simulink model "Cruise_Model_V16"  (R2024a)
settings: Solver=ode23t  StartTime=0.0  StopTime=t5(end)  RelTol=1e-3
values from neighbouring files (symbols this model uses):
  coefficients =     [UAM2.mat]    (also in VX4_cur.mat; VX4data.mat; alexisignoringme11UAM2.mat; alexisignoringme12.mat)
  idxf = [1 78 155 231 308 385 462 538 615 692 769 845 ... (70 elements, 1x70)]    [alexisignoringme.mat]    (also in alexisignoringme11UAM2.mat = [1 112 223 334 445 555 666 777 888 999 1001 1112 ... (50 ele; alexisignoringme12.mat = [1 54 106 159 211 264 316 369 421 474 526 579 ... (100 eleme; alexisignoringme13.mat = [1 54 106 159 211 264 316 369 421 474 526 579 ... (100 eleme; alexisignoringme14.mat = [1 500 999 1001 1500 1999 2001 2500 2999 3001 3500 3999 ... )
  Kpi = lqr(sys, Q, R)    [QRerr_LQI.m]    (also in alexisignoringme8.mat = [9.62344892608e-17 -1.21933000029e-16 1.4312558077e-15 29.45)
  missionruntime =     [alexisignoringme4.mat]    (also in alexisignoringme5.mat; alexisignoringme6.mat; alexisignoringme7.mat; alexisignoringme8.mat)
  q = 0.5*1.225*airflow.U^2    [VLMV3.m]    (also in VLMV3_modified.m = 0.5*1.225*airflow.U^2*Sref)
  Ut = [0 0 -4.89661324026e-08 0 0 -1504.57476188 -0.000428335964898 -1.57410795509e-09 3.42121377805e-06 0 0 0 ... (450 elements, 9x50)]    [alexisignoringme5.mat]    (also in alexisignoringme6.mat; alexisignoringme7.mat; alexisignoringme8.mat = [0 0 0 0 0 -1498.96331992 -4.41873387445e-05 -1.31180695462e)
  uvec = [0.1 3.42222222222 6.74444444444 10.0666666667 13.3888888889 16.7111111111 20.0333333333 23.3555555556 26.6777777778 30]    [alexisignoringme.mat]    (also in alexisignoringme4.mat; alexisignoringme5.mat; alexisignoringme6.mat; alexisignoringme7.mat)
  X = [0.00351660116596 0 -9.99999602467 0 0 0 2.75026701025e-08 -4.1982332666e-06 -1.5333765693e-08 0.000503097278932 0 -6.54626389426e-11 ... (630 elements, 9x5x14)]    [alexisignoringme.mat]    (also in alexisignoringme12.mat = [0.000256495736971 0 -9.99999647184 0 0 0 0 -3.73764411116e-; alexisignoringme13.mat = [0.00833666803911 0 -10.0000021435 0 0 0 0 7.14203458163e-06; alexisignoringme14.mat = [0.00833666803911 0 -10.0000021435 0 0 0 0 7.14203458163e-06; alexisignoringme4.mat = [0.00351658839646 0 -9.99999599468 0 0 0 2.7327442949e-09 -4)
  Xes = X(:,idx(4))    [QRerr_LQI.m]    (also in QRerr_p.m = X(:,idx(2)); alexisignoringme4.mat = [0.00351658839646 0 -9.99999599468 0 0 0 2.7327442949e-09 -4; alexisignoringme5.mat = [0 0 -1.11199998303 0 0 0 -1.38069247376e-09 1.48137256273e-; alexisignoringme6.mat = [0 0 -1.11199998303 0 0 0 -1.38069247376e-09 1.48137256273e-)
undefined symbols (not defined in the file or in its folder): F, Light, MIL, tl, VX4, xvec
libraries: slpidlib x14, aerolibwind2 x8, aerolibatmos2 x4, shared6dof x1
(part 3 of 3)

== system Cruise_Model_V16/Trim Solver and Actuation/Controller/Trim Solver/Back-calculation ==
  et : Inport
  Gain : Gain  Gain=2
  Transpose : Math  Operator=transpose
  Out1 : Outport
  wires:
  Gain/1 -> Transpose/1
  et/1 -> Gain/1
  Transpose/1 -> Out1/1

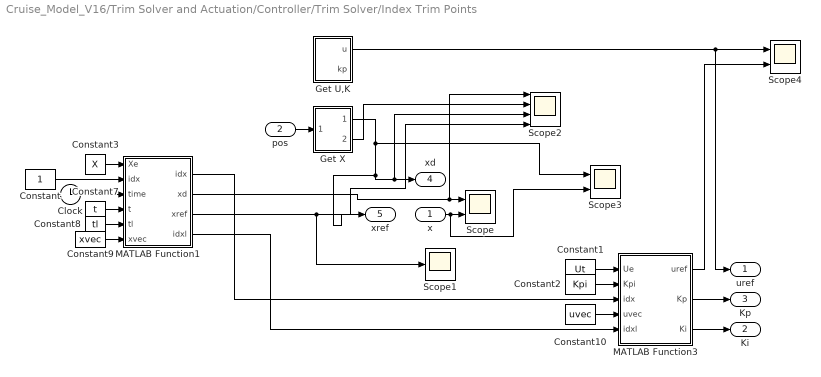
== system Cruise_Model_V16/Trim Solver and Actuation/Controller/Trim Solver/Index Trim Points ==
  x : Inport
  pos : Inport  Port=2
  Clock : Clock
  Constant : Constant
  Constant1 : Constant  Value=Ut
  Constant10 : Constant  Value=uvec
  Constant2 : Constant  Value=Kpi
  Constant3 : Constant  Value=X
  Constant7 : Constant  Value=t
  Constant8 : Constant  Value=tl
  Constant9 : Constant  Value=xvec
  Get U,K : Subsystem
  Get X : Subsystem
  MATLAB Function1 : MATLAB Function  InitFcn=load buses.mat  StartFcn=load buses.mat  TreatAsAtomicUnit=on  VariantControl=Choice
      settings: OpenFcn=load buses.mat
  MATLAB Function3 : MATLAB Function  InitFcn=load buses.mat  StartFcn=load buses.mat  TreatAsAtomicUnit=on  VariantControl=Choice
      settings: OpenFcn=load buses.mat
  Scope : Scope  NumInputPorts=2
  Scope1 : Scope
  Scope2 : Scope  NumInputPorts=4
  Scope3 : Scope  NumInputPorts=2
  Scope4 : Scope  NumInputPorts=2
  uref : Outport
  Ki : Outport  Port=2
  Kp : Outport  Port=3
  xd : Outport  Port=4
  xref : Outport  Port=5
  wires:
  Constant2/1 -> MATLAB Function3/2(Kpi)
  Constant1/1 -> MATLAB Function3/1(Ue)
  Constant3/1 -> MATLAB Function1/1(Xe)
  MATLAB Function3/1(uref) -> Scope4/2
  Constant8/1 -> MATLAB Function1/5(tl)
  Constant10/1 -> MATLAB Function3/4(uvec)
  MATLAB Function1/4(idxl) -> MATLAB Function3/5(idxl)
  MATLAB Function3/2(Kp) -> Kp/1
  Constant9/1 -> MATLAB Function1/6(xvec)
  Clock/1 -> MATLAB Function1/3(time)
  Constant7/1 -> MATLAB Function1/4(t)
  x/1 -> Scope3/2, Scope/2
  MATLAB Function3/3(Ki) -> Ki/1
  Constant/1 -> MATLAB Function1/2("idx ")
  MATLAB Function1/1(idx) -> MATLAB Function3/3(idx)
  MATLAB Function1/3(xref) -> Scope2/4, Scope1/1
  MATLAB Function1/2(xd) -> Scope2/1, Scope/1
  Get X/1(xref) -> xref/1, Scope2/3, xd/1, Scope3/1
  Get X/2(xd) -> Scope2/2
  Get U,K/1(u) -> uref/1, Scope4/1
  pos/1 -> Get X/1(pos)

== system Cruise_Model_V16/Trim Solver and Actuation/Controller/Trim Solver/Saturation1 ==
  In1 : Inport
  Constant : Constant  Value=0
  Demux3 : Demux  Outputs=9
  Mux : Mux  Inputs=9
  Saturation : Saturate  UpperLimit=0.55  LowerLimit=-0.55
  Saturation1 : Saturate  UpperLimit=0.55  LowerLimit=-0.55
  Saturation2 : Saturate  UpperLimit=0.55  LowerLimit=-0.55
  Saturation3 : Saturate  UpperLimit=1.6*max(abs(Ut(4,:)))  LowerLimit=0
  Saturation4 : Saturate  UpperLimit=0  LowerLimit=-1.6*max(abs(Ut(6,:)))
  Saturation5 : Saturate  UpperLimit=1.6*max(abs(Ut(6,:)))  LowerLimit=-1.6*max(abs(Ut(6,:)))
  Saturation6 : Saturate  UpperLimit=1.6*max(abs(Ut(6,:)))  LowerLimit=-1.6*max(abs(Ut(6,:)))
  Saturation7 : Saturate  UpperLimit=1.6*max(abs(Ut(6,:)))  LowerLimit=-1.6*max(abs(Ut(6,:)))
  Scope : Scope  NumInputPorts=2
  Out1 : Outport
  wires:
  Saturation7/1 -> Mux/9
  Saturation6/1 -> Mux/8
  Saturation5/1 -> Mux/7
  Saturation4/1 -> Mux/6
  Saturation3/1 -> Mux/4
  Saturation2/1 -> Mux/3
  Saturation1/1 -> Mux/2
  Saturation/1 -> Mux/1
  Demux3/9 -> Saturation7/1
  Constant/1 -> Mux/5
  Demux3/8 -> Saturation6/1
  Demux3/7 -> Saturation5/1
  Demux3/6 -> Saturation4/1
  Demux3/4 -> Saturation3/1
  In1/1 -> Demux3/1
  Mux/1 -> Out1/1
  Demux3/1 -> Saturation/1
  Demux3/2 -> Saturation1/1
  Demux3/3 -> Saturation2/1

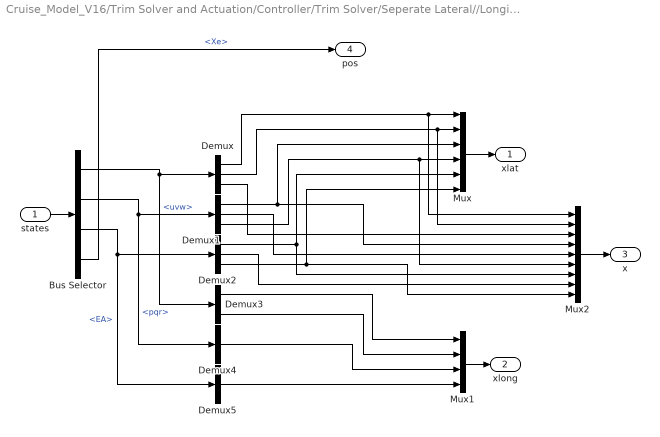
== system Cruise_Model_V16/Trim Solver and Actuation/Controller/Trim Solver/Seperate Lateral//Longitudinal ==
  states : Inport
  Bus Selector : BusSelector  OutputSignals=uvw,pqr,EA,Xe
  Demux{,1..5} (6 alike) : Demux  Outputs=3
  Mux : Mux  Inputs=6
  Mux1 : Mux
  Mux2 : Mux  Inputs=9
  xlat : Outport
  xlong : Outport  Port=2
  x : Outport  Port=3
  pos : Outport  Port=4
  wires:
  states/1 -> Bus Selector/1
  Mux/1 -> xlat/1
  Mux1/1 -> xlong/1
  Bus Selector/1 -> Demux/1, Demux3/1  "<uvw>"
  Bus Selector/2 -> Demux1/1, Demux4/1  "<pqr>"
  Bus Selector/3 -> Demux5/1, Demux2/1  "<EA>"
  Demux/1 -> Mux2/1, Mux/1
  Demux/2 -> Mux2/2, Mux/2
  Demux1/1 -> Mux2/4, Mux/3
  Demux1/3 -> Mux2/6, Mux/4
  Demux2/1 -> Mux2/7, Mux/5
  Demux2/3 -> Mux2/9, Mux/6
  Demux3/1 -> Mux1/1
  Demux3/3 -> Mux1/2
  Demux4/2 -> Mux1/3
  Demux5/2 -> Mux1/4
  Mux2/1 -> x/1
  Demux/3 -> Mux2/3
  Demux1/2 -> Mux2/5
  Demux2/2 -> Mux2/8
  Bus Selector/4 -> pos/1  "<Xe>"

== system Cruise_Model_V16/Trim Solver and Actuation/Controller/Trim Solver/State Passthr. ==
  In2 : Inport
  Demux3 : Demux  Outputs=9
  Mux3 : Mux  Inputs=6
  Terminator : Terminator
  Terminator1 : Terminator
  Terminator2 : Terminator
  Out4 : Outport
  wires:
  Demux3/1 -> Mux3/1
  Demux3/8 -> Mux3/5
  Demux3/7 -> Mux3/4
  Demux3/9 -> Mux3/6
  Demux3/3 -> Mux3/3
  Demux3/2 -> Mux3/2
  Mux3/1 -> Out4/1
  In2/1 -> Demux3/1
  Demux3/4 -> Terminator/1
  Demux3/5 -> Terminator1/1
  Demux3/6 -> Terminator2/1

== system Cruise_Model_V16/Trim Solver and Actuation/Controller/PID_GBDP_withThrust/Altitude Control Path/Step demand for testing ==
  In1 : Inport
  Mux1 : Mux  Inputs=2
  Scope2 : Scope
  Scope4 : Scope
  Step1 : Step  Time=60  Before=-500  After=-490  SampleTime=0
  Step2 : Step  Time=80  After=-10  SampleTime=0
  Step3 : Step  Time=120  After=20  SampleTime=0
  Step4 : Step  Time=120  After=20  SampleTime=0
  Sum : Sum  Inputs=++++
  To Workspace : ToWorkspace  VariableName=altitudeResponse  SaveFormat=Timeseries  SampleTime=-1
  Out1 : Outport
  wires:
  Step3/1 -> Sum/3
  Mux1/1 -> To Workspace/1, Scope4/1
  Sum/1 -> Out1/1, Mux1/1
  Step4/1 -> Sum/4
  Step1/1 -> Sum/1
  In1/1 -> Mux1/2, Scope2/1
  Step2/1 -> Sum/2

== system Cruise_Model_V16/Trim Solver and Actuation/Controller/PID_GBDP_withThrust/Course Angle Control Path/Step demand for testing2 ==
  Va : Inport
  Mux1 : Mux  Inputs=2
  Scope2 : Scope
  Scope4 : Scope
  Step1 : Step  Time=60  Before=0.1  After=0.2  SampleTime=0
  Step2 : Step  Time=80  After=-0.4  SampleTime=0
  Step3 : Step  Time=120  After=-0.2  SampleTime=0
  Step4 : Step  Time=100  After=0.6  SampleTime=0
  Step5 : Step  Time=140  After=-0.4  SampleTime=0
  Sum : Sum  Inputs=+++++
  To Workspace : ToWorkspace  VariableName=headingAngleResponse  SaveFormat=Timeseries  SampleTime=-1
  Out1 : Outport
  wires:
  Step5/1 -> Sum/5
  Step3/1 -> Sum/3
  Mux1/1 -> To Workspace/1, Scope4/1
  Sum/1 -> Out1/1, Mux1/1
  Step4/1 -> Sum/4
  Step1/1 -> Sum/1
  Va/1 -> Mux1/2, Scope2/1
  Step2/1 -> Sum/2

== system Cruise_Model_V16/Trim Solver and Actuation/Controller/PID_GBDP_withThrust/Subsystem/Step demand for testing1 ==
  Va : Inport
  Mux1 : Mux  Inputs=2
  Scope2 : Scope
  Scope4 : Scope
  Step1 : Step  Time=60  Before=25  After=31  SampleTime=0
  Step2 : Step  Time=80  After=-3  SampleTime=0
  Step3 : Step  Time=120  After=-5  SampleTime=0
  Step4 : Step  Time=100  After=8  SampleTime=0
  Step5 : Step  Time=140  After=-2  SampleTime=0
  Sum : Sum  Inputs=+++++
  To Workspace : ToWorkspace  VariableName=airspeedResponse  SaveFormat=Timeseries  SampleTime=-1
  Out1 : Outport
  wires:
  Step2/1 -> Sum/2
  Va/1 -> Scope2/1, Mux1/2
  Step1/1 -> Sum/1
  Step4/1 -> Sum/4
  Sum/1 -> Mux1/1, Out1/1
  Mux1/1 -> Scope4/1, To Workspace/1
  Step3/1 -> Sum/3
  Step5/1 -> Sum/5

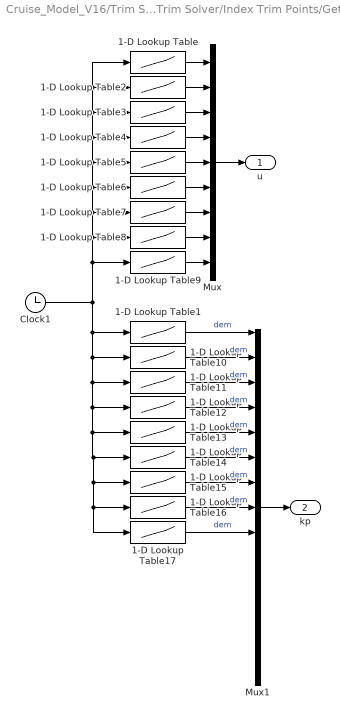
== system Cruise_Model_V16/Trim Solver and Actuation/Controller/Trim Solver/Index Trim Points/Get U,K ==
  1-D Lookup Table : Lookup_n-D  NumberOfTableDimensions=1  BreakpointsForDimension1=t  Table=Ut(1,:)  InternalRulePriority=Speed  RndMeth=Simplest
  1-D Lookup Table1 : Lookup_n-D  NumberOfTableDimensions=1  BreakpointsForDimension1=t(1:end-1)  Table=X(1,2:end)  InternalRulePriority=Speed  RndMeth=Simplest
  1-D Lookup Table10 : Lookup_n-D  NumberOfTableDimensions=1  BreakpointsForDimension1=t(1:end-1)  Table=X(2,2:end)  InternalRulePriority=Speed  RndMeth=Simplest
  1-D Lookup Table11 : Lookup_n-D  NumberOfTableDimensions=1  BreakpointsForDimension1=t(1:end-1)  Table=X(3,2:end)  InternalRulePriority=Speed  RndMeth=Simplest
  1-D Lookup Table12 : Lookup_n-D  NumberOfTableDimensions=1  BreakpointsForDimension1=t(1:end-1)  Table=X(4,2:end)  InternalRulePriority=Speed  RndMeth=Simplest
  1-D Lookup Table13 : Lookup_n-D  NumberOfTableDimensions=1  BreakpointsForDimension1=t(1:end-1)  Table=X(5,2:end)  InternalRulePriority=Speed  RndMeth=Simplest
  1-D Lookup Table14 : Lookup_n-D  NumberOfTableDimensions=1  BreakpointsForDimension1=t(1:end-1)  Table=X(6,2:end)  InternalRulePriority=Speed  RndMeth=Simplest
  1-D Lookup Table15 : Lookup_n-D  NumberOfTableDimensions=1  BreakpointsForDimension1=t(1:end-1)  Table=X(7,2:end)  InternalRulePriority=Speed  RndMeth=Simplest
  1-D Lookup Table16 : Lookup_n-D  NumberOfTableDimensions=1  BreakpointsForDimension1=t(1:end-1)  Table=X(8,2:end)  InternalRulePriority=Speed  RndMeth=Simplest
  1-D Lookup Table17 : Lookup_n-D  NumberOfTableDimensions=1  BreakpointsForDimension1=t(1:end-1)  Table=X(9,2:end)  InternalRulePriority=Speed  RndMeth=Simplest
  1-D Lookup Table2 : Lookup_n-D  NumberOfTableDimensions=1  BreakpointsForDimension1=t  Table=Ut(2,:)  InternalRulePriority=Speed  RndMeth=Simplest
  1-D Lookup Table3 : Lookup_n-D  NumberOfTableDimensions=1  BreakpointsForDimension1=t  Table=Ut(3,:)  InternalRulePriority=Speed  RndMeth=Simplest
  1-D Lookup Table4 : Lookup_n-D  NumberOfTableDimensions=1  BreakpointsForDimension1=t  Table=Ut(4,:)  InternalRulePriority=Speed  RndMeth=Simplest
  1-D Lookup Table5 : Lookup_n-D  NumberOfTableDimensions=1  BreakpointsForDimension1=t  Table=Ut(5,:)  InternalRulePriority=Speed  RndMeth=Simplest
  1-D Lookup Table6 : Lookup_n-D  NumberOfTableDimensions=1  BreakpointsForDimension1=t  Table=Ut(6,:)  InternalRulePriority=Speed  RndMeth=Simplest
  1-D Lookup Table7 : Lookup_n-D  NumberOfTableDimensions=1  BreakpointsForDimension1=t  Table=Ut(7,:)  InternalRulePriority=Speed  RndMeth=Simplest
  1-D Lookup Table8 : Lookup_n-D  NumberOfTableDimensions=1  BreakpointsForDimension1=t  Table=Ut(8,:)  InternalRulePriority=Speed  RndMeth=Simplest
  1-D Lookup Table9 : Lookup_n-D  NumberOfTableDimensions=1  BreakpointsForDimension1=t  Table=Ut(9,:)  InternalRulePriority=Speed  RndMeth=Simplest
  Clock1 : Clock
  Mux : Mux  Inputs=9
  Mux1 : Mux  Inputs=15
  u : Outport
  kp : Outport  Port=2
  wires:
  1-D Lookup Table17/1 -> Mux1/9  "dem"
  1-D Lookup Table16/1 -> Mux1/8  "dem"
  1-D Lookup Table15/1 -> Mux1/7  "dem"
  1-D Lookup Table14/1 -> Mux1/6  "dem"
  1-D Lookup Table13/1 -> Mux1/5  "dem"
  1-D Lookup Table12/1 -> Mux1/4  "dem"
  1-D Lookup Table11/1 -> Mux1/3  "dem"
  1-D Lookup Table10/1 -> Mux1/2  "dem"
  1-D Lookup Table1/1 -> Mux1/1  "dem"
  Mux1/1 -> kp/1
  1-D Lookup Table9/1 -> Mux/9
  1-D Lookup Table8/1 -> Mux/8
  1-D Lookup Table7/1 -> Mux/7
  1-D Lookup Table6/1 -> Mux/6
  1-D Lookup Table5/1 -> Mux/5
  1-D Lookup Table4/1 -> Mux/4
  1-D Lookup Table3/1 -> Mux/3
  Clock1/1 -> 1-D Lookup Table12/1, 1-D Lookup Table13/1, 1-D Lookup Table14/1, 1-D Lookup Table15/1, 1-D Lookup Table16/1, 1-D Lookup Table17/1, 1-D Lookup Table11/1, 1-D Lookup Table10/1, 1-D Lookup Table1/1, 1-D Lookup Table9/1, 1-D Lookup Table8/1, 1-D Lookup Table7/1, 1-D Lookup Table6/1, 1-D Lookup Table5/1, 1-D Lookup Table4/1, 1-D Lookup Table3/1, 1-D Lookup Table2/1, 1-D Lookup Table/1
  1-D Lookup Table2/1 -> Mux/2
  Mux/1 -> u/1
  1-D Lookup Table/1 -> Mux/1

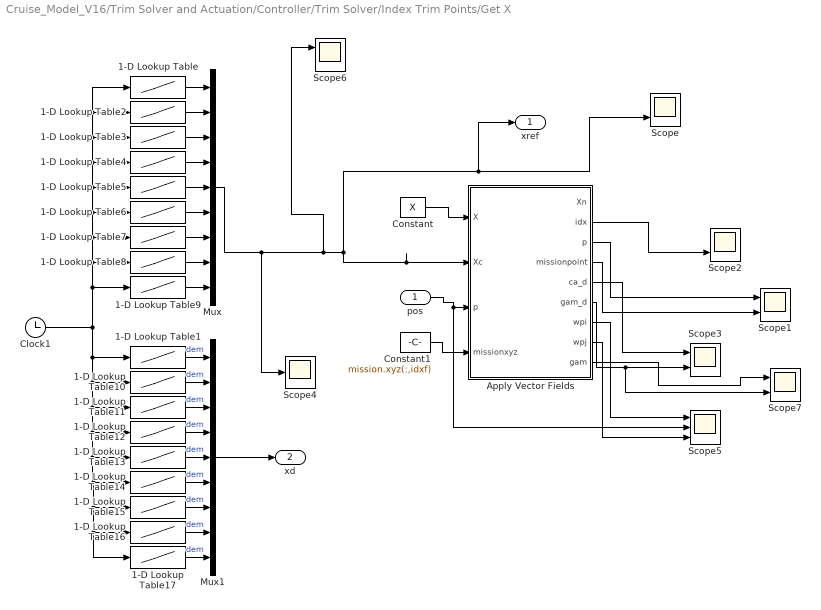
== system Cruise_Model_V16/Trim Solver and Actuation/Controller/Trim Solver/Index Trim Points/Get X ==
  pos : Inport
  1-D Lookup Table : Lookup_n-D  NumberOfTableDimensions=1  BreakpointsForDimension1=t  Table=X(1,:)  InternalRulePriority=Speed  RndMeth=Simplest
  1-D Lookup Table1 : Lookup_n-D  NumberOfTableDimensions=1  BreakpointsForDimension1=t(1:end-1)  Table=X(1,2:end)  InternalRulePriority=Speed  RndMeth=Simplest
  1-D Lookup Table10 : Lookup_n-D  NumberOfTableDimensions=1  BreakpointsForDimension1=t(1:end-1)  Table=X(2,2:end)  InternalRulePriority=Speed  RndMeth=Simplest
  1-D Lookup Table11 : Lookup_n-D  NumberOfTableDimensions=1  BreakpointsForDimension1=t(1:end-1)  Table=X(3,2:end)  InternalRulePriority=Speed  RndMeth=Simplest
  1-D Lookup Table12 : Lookup_n-D  NumberOfTableDimensions=1  BreakpointsForDimension1=t(1:end-1)  Table=X(4,2:end)  InternalRulePriority=Speed  RndMeth=Simplest
  1-D Lookup Table13 : Lookup_n-D  NumberOfTableDimensions=1  BreakpointsForDimension1=t(1:end-1)  Table=X(5,2:end)  InternalRulePriority=Speed  RndMeth=Simplest
  1-D Lookup Table14 : Lookup_n-D  NumberOfTableDimensions=1  BreakpointsForDimension1=t(1:end-1)  Table=X(6,2:end)  InternalRulePriority=Speed  RndMeth=Simplest
  1-D Lookup Table15 : Lookup_n-D  NumberOfTableDimensions=1  BreakpointsForDimension1=t(1:end-1)  Table=X(7,2:end)  InternalRulePriority=Speed  RndMeth=Simplest
  1-D Lookup Table16 : Lookup_n-D  NumberOfTableDimensions=1  BreakpointsForDimension1=t(1:end-1)  Table=X(8,2:end)  InternalRulePriority=Speed  RndMeth=Simplest
  1-D Lookup Table17 : Lookup_n-D  NumberOfTableDimensions=1  BreakpointsForDimension1=t(1:end-1)  Table=X(9,2:end)  InternalRulePriority=Speed  RndMeth=Simplest
  1-D Lookup Table2 : Lookup_n-D  NumberOfTableDimensions=1  BreakpointsForDimension1=t  Table=X(2,:)  InternalRulePriority=Speed  RndMeth=Simplest
  1-D Lookup Table3 : Lookup_n-D  NumberOfTableDimensions=1  BreakpointsForDimension1=t  Table=X(3,:)  InternalRulePriority=Speed  RndMeth=Simplest
  1-D Lookup Table4 : Lookup_n-D  NumberOfTableDimensions=1  BreakpointsForDimension1=t  Table=X(4,:)  InternalRulePriority=Speed  RndMeth=Simplest
  1-D Lookup Table5 : Lookup_n-D  NumberOfTableDimensions=1  BreakpointsForDimension1=t  Table=X(5,:)  InternalRulePriority=Speed  RndMeth=Simplest
  1-D Lookup Table6 : Lookup_n-D  NumberOfTableDimensions=1  BreakpointsForDimension1=t  Table=X(6,:)  InternalRulePriority=Speed  RndMeth=Simplest
  1-D Lookup Table7 : Lookup_n-D  NumberOfTableDimensions=1  BreakpointsForDimension1=t  Table=X(7,:)  InternalRulePriority=Speed  RndMeth=Simplest
  1-D Lookup Table8 : Lookup_n-D  NumberOfTableDimensions=1  BreakpointsForDimension1=t  Table=X(8,:)  InternalRulePriority=Speed  RndMeth=Simplest
  1-D Lookup Table9 : Lookup_n-D  NumberOfTableDimensions=1  BreakpointsForDimension1=t  Table=X(9,:)  InternalRulePriority=Speed  RndMeth=Simplest
  Apply Vector Fields : MATLAB Function  TreatAsAtomicUnit=on
  Clock1 : Clock
  Constant : Constant  Value=X
  Constant1 : Constant  Value=mission.xyz(:,idxf)
  Mux : Mux  Inputs=9
  Mux1 : Mux  Inputs=9
  Scope{,1..3,6..7} (6 alike) : Scope  NumInputPorts=2
  Scope4 : Scope
  Scope5 : Scope  NumInputPorts=3
  xref : Outport
  xd : Outport  Port=2
  wires:
  1-D Lookup Table/1 -> Mux/1
  Mux/1 -> Scope6/1, Apply Vector Fields/2(Xc), xref/1, Scope/2, Scope4/1
  1-D Lookup Table2/1 -> Mux/2
  Clock1/1 -> 1-D Lookup Table/1, 1-D Lookup Table2/1, 1-D Lookup Table3/1, 1-D Lookup Table4/1, 1-D Lookup Table5/1, 1-D Lookup Table6/1, 1-D Lookup Table7/1, 1-D Lookup Table8/1, 1-D Lookup Table9/1, 1-D Lookup Table1/1, 1-D Lookup Table10/1, 1-D Lookup Table11/1, 1-D Lookup Table17/1, 1-D Lookup Table16/1, 1-D Lookup Table15/1, 1-D Lookup Table14/1, 1-D Lookup Table13/1, 1-D Lookup Table12/1
  1-D Lookup Table3/1 -> Mux/3
  1-D Lookup Table4/1 -> Mux/4
  1-D Lookup Table5/1 -> Mux/5
  1-D Lookup Table6/1 -> Mux/6
  1-D Lookup Table7/1 -> Mux/7
  1-D Lookup Table8/1 -> Mux/8
  1-D Lookup Table9/1 -> Mux/9
  1-D Lookup Table1/1 -> Mux1/1  "dem"
  1-D Lookup Table10/1 -> Mux1/2  "dem"
  1-D Lookup Table11/1 -> Mux1/3  "dem"
  1-D Lookup Table12/1 -> Mux1/4  "dem"
  1-D Lookup Table13/1 -> Mux1/5  "dem"
  1-D Lookup Table14/1 -> Mux1/6  "dem"
  1-D Lookup Table15/1 -> Mux1/7  "dem"
  1-D Lookup Table16/1 -> Mux1/8  "dem"
  1-D Lookup Table17/1 -> Mux1/9  "dem"
  Constant/1 -> Apply Vector Fields/1(X)
  pos/1 -> Scope5/2, Apply Vector Fields/3("p ")
  Constant1/1 -> Apply Vector Fields/4(missionxyz)
  Apply Vector Fields/3(p) -> Scope1/1
  Apply Vector Fields/4(missionpoint) -> Scope1/2
  Mux1/1 -> xd/1
  Apply Vector Fields/2(idx) -> Scope2/2
  Apply Vector Fields/5(ca_d) -> Scope3/1
  Apply Vector Fields/7(wpi) -> Scope5/1
  Apply Vector Fields/8(wpj) -> Scope5/3
  Apply Vector Fields/9(gam) -> Scope7/1
  Apply Vector Fields/6(gam_d) -> Scope7/2, Scope3/2

== matlab function Cruise_Model_V16/Trim Solver and Actuation/Controller/Trim Solver/Index Trim Points/MATLAB Function3 ==
  data: uref output; Ue input; Kpi input; idx input; Kp output; uvec input; idxl input; Ki output
function [uref, Kp, Ki]  = fcn(Ue, Kpi, idx, uvec, idxl)

% uref = Ue(:,idx);
uref = uvec(:,idxl);
if idx < 100
    Kp = -Kpi(:,1:9,idx);
    Ki = -Kpi(:,10:15,idx);
else
    Kp = -Kpi(:,1:9,idx);
    Ki = -Kpi(:,10:15,idx);
end

== matlab function Cruise_Model_V16/Trim Solver and Actuation/Controller/Trim Solver/Index Trim Points/Get X/Apply Vector Fields ==
  data: Xn output; X input; Xc input; p input; idx output; missionxyz input; p output; missionpoint output; ca_d output; gam_d output; wpi output; wpj output; gam output
function [Xn, idx, p, missionpoint, ca_d, gam_d, wpi, wpj, gam] = fcn(X, Xc, p, missionxyz)

[Xn, idx, gam] = calcStateVF(missionxyz.*[1 1 -1]', X, Xc, p, 0.2, 0.2, 0.3, 0.3);
missionpoint = missionxyz(:,idx).*[1 1 -1]';


[ca_d, gam_d, wpi, wpj] = createDemandVecVF(missionxyz.*[1 1 -1]', p, 0.2, 0.2, 0.3, 0.3);

== matlab function Cruise_Model_V16/Aircraft Dynamics/Aerodynamic Forces and Moments/MATLAB Function ==
  data: Fb output; Mcg output; coeff input Bus: coeff; u input; alpha input; beta input; V input; rho input; X input; refGeo parameter; m parameter; thrust input; cg parameter
function [Fb,Mcg] = aeroDyn(coeff, u, alpha, beta, V, rho, X, refGeo, m, thrust, cg)
% Function aeroDyn simulates ....

%% Setting up intermediate variables
b = refGeo.bref;
S = refGeo.Sref;
c = refGeo.cref;

Q = 0.5*rho*V^2; % Dynamic pressure Q

ndc = c/(2*V);
ndb = b/(2*V);

%% Seperating vectors (BFR)
uvw = X(1:3); % Translational velocity vector
pqr = X(4:6); % Angular velocity vector
EA = X(7:end);

%% Handle Stall

%% Non-dimensional Aerodynamic Force Coefficients
% In wind axis
% Lift
CL = applyDeriv(coeff.CL0, coeff.CLa, coeff.CLb, coeff.CLn, 0, coeff.CLq, 0, u, alpha, beta, pqr, ndc);

% Drag 
CD = applyDeriv(coeff.CD0, coeff.CDa, coeff.CDb, coeff.CDn, 0, 0, 0, u, alpha, beta, pqr, ndc);

% Sideforce
CY = applyDeriv(0, coeff.CYa, coeff.CYb, coeff.CYn, coeff.CYp, 0, coeff.CYr, u, alpha, beta, pqr, ndb);

if abs(alpha) > 14.5*(pi/180)
    CL = 0;
    CD = coeff.CD0;
    CY = 0;
end

%% Rotate wind to body
Faw = [-max(CD,0); CY; -CL].*Q*S; % Force vector in the stability frame

Rwb = [cos(alpha)*cos(beta), -cos(alpha)*sin(beta), -sin(alpha);  
       sin(beta)           ,  cos(beta)           ,  0         ; 
       cos(beta)*sin(alpha), -sin(alpha)*sin(beta),  cos(alpha)];

Fab = Rwb*Faw; % aerodynamic force on body

%% Aerodynamic Moment about CG
% In Fb, with moments taken about the centre of gravity

% Roll
Cl = applyDeriv(0, coeff.Cla, coeff.Clb, coeff.Cln, coeff.Clp, 0, coeff.Clr, u, alpha, beta, pqr, ndb);

% Pitch
Cm = applyDeriv(coeff.Cm0, coeff.Cma, coeff.Cmb, coeff.Cmn, 0, coeff.Cmq, 0, u, alpha, beta, pqr, ndc);

% Yaw
Cn = applyDeriv(0, coeff.Cna, coeff.Cnb, coeff.Cnn, coeff.Cnp, 0, coeff.Cnr, u, alpha, beta, pqr, ndb);

if abs(alpha) > 20*(pi/180)
    Cm = 0;
    Cn = 0;
    Cl = 0;
end

Ma = [b*Cl; c*Cm; b*Cn].*Q*S;

%% Propulsion Effects
% Moment and forces induced by throttle
FTb = u(4:6);
MTcg = u(7:9);

% Gravity Effects
Fgb = [-9.81*sin(X(8))          ; % Body frame
        9.81*cos(X(8))*sin(X(7));
        9.81*cos(X(8))*cos(X(7))]*m; % ASSUMPTION: Constant Mass

%% Out
Rbe = body2earth(X(7), X(8), X(9));

Fb = FTb + Fgb + Fab;
Mcg = MTcg + Ma;

forces = [FTb; Fgb; Fab; Rbe*Fb];
aero = [CL; CD; Cm];
uvw_e = Rbe*X(1:3);

end

%% Extra functions

function C = applyDeriv(C0, Ca, Cb, Cn, Cp, Cq, Cr, u, alpha, beta, pqr, nd)
% function applyDeriv calculates the coefficient C from the derivatives C0,
% Ca, Cb, Cn wrt 0, alpha, beta and control (n), respectively.

    C_nc = C0 + Ca*alpha + Cb*beta + Cp*pqr(1)*nd + Cq*pqr(2)*nd + Cr*pqr(3)*nd; % lift coefficient no control
    
    C_c = (Cn.*u(1:length(Cn)))';

    C = C_nc + sum(C_c);

end

== matlab function Cruise_Model_V16/Trim Solver and Actuation/Controller/Trim Solver/Index Trim Points/MATLAB Function1 ==
  data: idx output; Xe input; idx input; mission parameter; xd output; xref output; time input; t input; tl input; xvec input; idxl output
function [idx, xd, xref, idxl] = fcn(Xe, idx, mission, time, t, tl, xvec)

[~, idx] = max(t(t <= time));
[~, idxl] = max(tl(tl <= time));
% 
xd = xvec(:,idxl);
xref = xvec(:,idxl);
% xref = Xe(:,idx);

% xd = Xe(:,idx+1);
